simulink model "SPWH"  (R2022a)
settings: Solver=VariableStepAuto  StartTime=0.0  StopTime=84600  RelTol=1e-3
model workspace (MAT data in the model file):
  A = 10
  Eff = 0.8
  a = 5
  b = 5
undefined symbols (not defined in the file): B1, B49, csv, F1, F49, G1, G49, WeatherInput
libraries: slpidlib x2
settings Model: Creator=harry  LastModifiedBy=harry

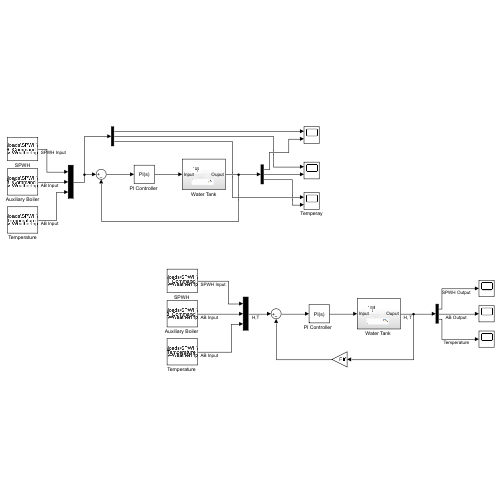
[thumbnail: Simulink's stored preview of the top-level diagram]
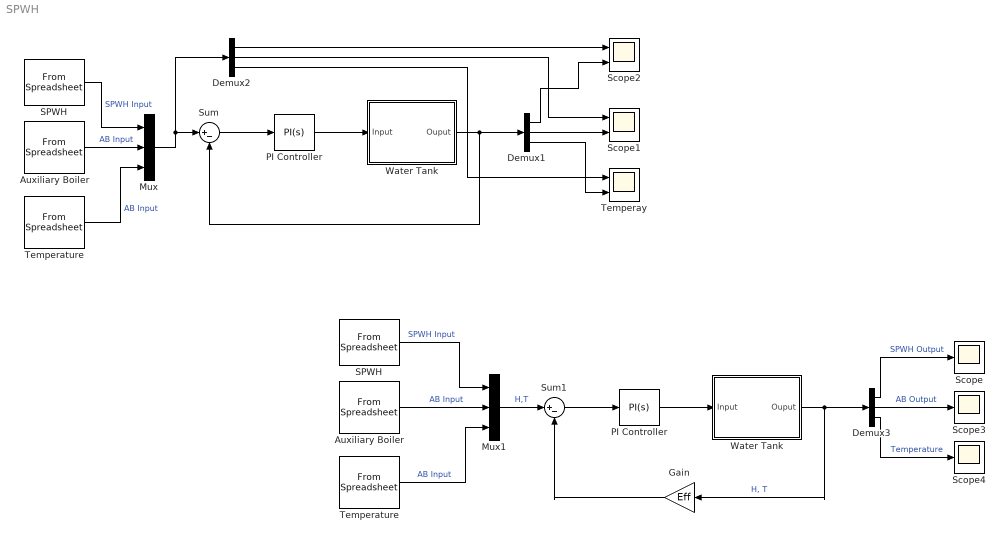
== system SPWH ==
  Auxiliary Boiler : FromSpreadsheet  FileName=C:\Users\harry\Downloads\SPWH\profiler-analyzer.xlsx  SheetName=csv-WeatherInput  Range=B1:B49,E1:E49
  "Auxiliary Boiler " : FromSpreadsheet  FileName=C:\Users\harry\Downloads\SPWH\profiler-analyzer.xlsx  SheetName=csv-WeatherInput  Range=B1:B49,E1:E49
  Demux1 : Demux  Outputs=3
  Demux2 : Demux  Outputs=3
  Demux3 : Demux  Outputs=3
  Gain : Gain  Gain=Eff
  Mux : Mux  Inputs=3
  Mux1 : Mux  Inputs=3
  "PI Controller " : slpidlib/PID Controller  Controller=PI  Form=Parallel  TimeDomain=Continuous-time  UseExternalTs=off  SampleTime=-1  IntegratorMethod=Forward Euler  FilterMethod=Forward Euler  ControllerParametersSource=internal  P=100  I=100  UseKiTs=off  D=0  N=100  UseFilter=on  TunerSelectOption=Transfer Function Based (PID Tuner App)  InitialConditionSource=internal  InitialConditionForIntegrator=0  InitialConditionForFilter=0  DifferentiatorICPrevScaledInput=0  ExternalReset=none  TrackingMode=off  Kt=1  LimitOutput=off  SatLimitsSource=internal  UpperSaturationLimit=inf  LowerSaturationLimit=-inf  LinearizeAsGain=on  AntiWindupMode=none  Kb=1  POutMin=[]  POutMax=[]  IOutMin=[]  IOutMax=[]  DOutMin=[]  DOutMax=[]  NOutMin=[]  NOutMax=[]  SumOutMin=[]  SumOutMax=[]  SaturationOutMin=[]  SaturationOutMax=[]  PParamMin=[]  PParamMax=[]  IParamMin=[]  IParamMax=[]  DParamMin=[]  DParamMax=[]  NParamMin=[]  NParamMax=[]  KbParamMin=[]  KbParamMax=[]  KtParamMin=[]  KtParamMax=[]  KbOutMin=[]  KbOutMax=[]  KtOutMin=[]  KtOutMax=[]  IntegratorOutMin=[]  IntegratorOutMax=[]  FilterOutMin=[]  FilterOutMax=[]  SumI1OutMin=[]  SumI1OutMax=[]  SumI2OutMin=[]  SumI2OutMax=[]  SumI3OutMin=[]  SumI3OutMax=[]  SumI4OutMin=[]  SumI4OutMax=[]  SumDOutMin=[]  SumDOutMax=[]  DifferentiatorOutMin=[]  DifferentiatorOutMax=[]  FilterDiffOutCoefMin=[]  FilterDiffOutCoefMax=[]  ReciprocalOutMin=[]  ReciprocalOutMax=[]  SumDenOutMin=[]  SumDenOutMax=[]  SumNumOutMin=[]  SumNumOutMax=[]  DivideOutMin=[]  DivideOutMax=[]  UdiffTsProdOutMin=[]  UdiffTsProdOutMax=[]  NTsProdOutMin=[]  NTsProdOutMax=[]  UintegralTsProdOutMin=[]  UintegralTsProdOutMax=[]  UngainTsProdOutMin=[]  UngainTsProdOutMax=[]  IntegratorContinuousStateAttributes=''  IntegratorStateMustResolveToSignalObject=off  IntegratorRTWStateStorageClass=Auto  FilterContinuousStateAttributes=''  FilterStateMustResolveToSignalObject=off  FilterRTWStateStorageClass=Auto  ParallelPVariant=InternalParameters  IdealPVariant=Disabled  IVariant=InternalParameters  DVariant=Disabled  IntegratorVariant=Continuous  SatVariant=Disabled  AWVariant=Passthrough  PCopyVariant=Disabled  TRVariant=Disabled  FdbkBlocksVariant=Forward  IdealPFdbkVariant=Disabled  SatFdbkVariant=Disabled  DerivativeFilterVariant=Disabled  NVariant=Disabled  NCopyVariant=Disabled_SignalSpec  FilterICVariant=Disabled  IntegratorICVariant=InternalICs  ExternalResetVariant=Disabled  TRSumVariant=Passthrough  SumFdbkVariant=Disabled  SumVariant=Sum_PI  TsampFilterVariant=InternalTs  TsampNgainVariant=Passthrough  TsampIntegralVariant=Passthrough  ExternalSaturationOutDataTypeStr=Inherit: Same as second input  aMode=0
  "PI Controller  " : slpidlib/PID Controller  Controller=PI  Form=Parallel  TimeDomain=Continuous-time  UseExternalTs=off  SampleTime=-1  IntegratorMethod=Forward Euler  FilterMethod=Forward Euler  ControllerParametersSource=internal  P=1  I=1  UseKiTs=off  D=0  N=100  UseFilter=on  TunerSelectOption=Transfer Function Based (PID Tuner App)  InitialConditionSource=internal  InitialConditionForIntegrator=0  InitialConditionForFilter=0  DifferentiatorICPrevScaledInput=0  ExternalReset=none  TrackingMode=off  Kt=1  LimitOutput=off  SatLimitsSource=internal  UpperSaturationLimit=inf  LowerSaturationLimit=-inf  LinearizeAsGain=on  AntiWindupMode=none  Kb=1  POutMin=[]  POutMax=[]  IOutMin=[]  IOutMax=[]  DOutMin=[]  DOutMax=[]  NOutMin=[]  NOutMax=[]  SumOutMin=[]  SumOutMax=[]  SaturationOutMin=[]  SaturationOutMax=[]  PParamMin=[]  PParamMax=[]  IParamMin=[]  IParamMax=[]  DParamMin=[]  DParamMax=[]  NParamMin=[]  NParamMax=[]  KbParamMin=[]  KbParamMax=[]  KtParamMin=[]  KtParamMax=[]  KbOutMin=[]  KbOutMax=[]  KtOutMin=[]  KtOutMax=[]  IntegratorOutMin=[]  IntegratorOutMax=[]  FilterOutMin=[]  FilterOutMax=[]  SumI1OutMin=[]  SumI1OutMax=[]  SumI2OutMin=[]  SumI2OutMax=[]  SumI3OutMin=[]  SumI3OutMax=[]  SumI4OutMin=[]  SumI4OutMax=[]  SumDOutMin=[]  SumDOutMax=[]  DifferentiatorOutMin=[]  DifferentiatorOutMax=[]  FilterDiffOutCoefMin=[]  FilterDiffOutCoefMax=[]  ReciprocalOutMin=[]  ReciprocalOutMax=[]  SumDenOutMin=[]  SumDenOutMax=[]  SumNumOutMin=[]  SumNumOutMax=[]  DivideOutMin=[]  DivideOutMax=[]  UdiffTsProdOutMin=[]  UdiffTsProdOutMax=[]  NTsProdOutMin=[]  NTsProdOutMax=[]  UintegralTsProdOutMin=[]  UintegralTsProdOutMax=[]  UngainTsProdOutMin=[]  UngainTsProdOutMax=[]  IntegratorContinuousStateAttributes=''  IntegratorStateMustResolveToSignalObject=off  IntegratorRTWStateStorageClass=Auto  FilterContinuousStateAttributes=''  FilterStateMustResolveToSignalObject=off  FilterRTWStateStorageClass=Auto  ParallelPVariant=InternalParameters  IdealPVariant=Disabled  IVariant=InternalParameters  DVariant=Disabled  IntegratorVariant=Continuous  SatVariant=Disabled  AWVariant=Passthrough  PCopyVariant=Disabled  TRVariant=Disabled  FdbkBlocksVariant=Forward  IdealPFdbkVariant=Disabled  SatFdbkVariant=Disabled  DerivativeFilterVariant=Disabled  NVariant=Disabled  NCopyVariant=Disabled_SignalSpec  FilterICVariant=Disabled  IntegratorICVariant=InternalICs  ExternalResetVariant=Disabled  TRSumVariant=Passthrough  SumFdbkVariant=Disabled  SumVariant=Sum_PI  TsampFilterVariant=InternalTs  TsampNgainVariant=Passthrough  TsampIntegralVariant=Passthrough  ExternalSaturationOutDataTypeStr=Inherit: Same as second input  aMode=0
  SPWH : FromSpreadsheet  FileName=C:\Users\harry\Downloads\SPWH\profiler-analyzer.xlsx  SheetName=csv-WeatherInput  Range=B1:B49,F1:F49
  "SPWH " : FromSpreadsheet  FileName=C:\Users\harry\Downloads\SPWH\profiler-analyzer.xlsx  SheetName=csv-WeatherInput  Range=B1:B49,F1:F49
  Scope : Scope
  Scope1 : Scope  NumInputPorts=2
  Scope2 : Scope  NumInputPorts=2
  Scope3 : Scope
  Scope4 : Scope
  Sum : Sum  Inputs=|+-
  Sum1 : Sum  Inputs=|+-
  Temperature : FromSpreadsheet  FileName=C:\Users\harry\Downloads\SPWH\profiler-analyzer.xlsx  SheetName=csv-WeatherInput  Range=B1:B49,G1:G49
  "Temperature " : FromSpreadsheet  FileName=C:\Users\harry\Downloads\SPWH\profiler-analyzer.xlsx  SheetName=csv-WeatherInput  Range=B1:B49,G1:G49
  Temperay : Scope  NumInputPorts=2
  Water Tank : Subsystem
  "Water Tank " : Subsystem
  wires:
  Water Tank/1(Ouput) -> Demux1/1, Sum/2
  Auxiliary Boiler/1 -> Mux/2  "AB Input"
  SPWH/1 -> Mux/1  "SPWH Input"
  Mux/1 -> Demux2/1, Sum/1
  Sum/1 -> "PI Controller "/1
  "PI Controller "/1 -> Water Tank/1("Input ")
  Demux1/1 -> Scope2/2
  Demux1/2 -> Scope1/2
  Demux2/1 -> Scope2/1
  Demux2/3 -> Temperay/1
  Temperature/1 -> Mux/3  "AB Input"
  Demux2/2 -> Scope1/1
  Demux1/3 -> Temperay/2
  Demux3/3 -> Scope4/1  "Temperature"
  Sum1/1 -> "PI Controller  "/1
  "Water Tank "/1(Ouput) -> Demux3/1, Gain/1  "H, T"
  "PI Controller  "/1 -> "Water Tank "/1("Input ")
  "Temperature "/1 -> Mux1/3  "AB Input"
  Demux3/2 -> Scope3/1  "AB Output"
  Demux3/1 -> Scope/1  "SPWH Output"
  "Auxiliary Boiler "/1 -> Mux1/2  "AB Input"
  "SPWH "/1 -> Mux1/1  "SPWH Input"
  Mux1/1 -> Sum1/1  "H,T"
  Gain/1 -> Sum1/2

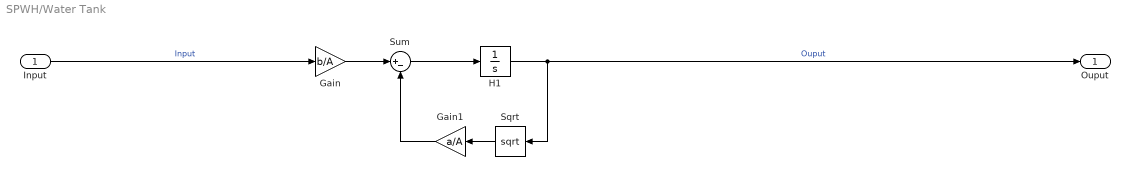
== system SPWH/Water Tank ==
  "Input " : Inport
  Gain : Gain  Gain=b/A
  Gain1 : Gain  Gain=a/A
  H1 : Integrator  InitialCondition=3  LimitOutput=on  LowerSaturationLimit=0
  Sqrt : Sqrt
  Sum : Sum  Inputs=|+-
  Ouput : Outport
  wires:
  Gain1/1 -> Sum/2
  "Input "/1 -> Gain/1  "Input"
  H1/1 -> Sqrt/1, Ouput/1  "Ouput"
  Gain/1 -> Sum/1
  Sum/1 -> H1/1
  Sqrt/1 -> Gain1/1

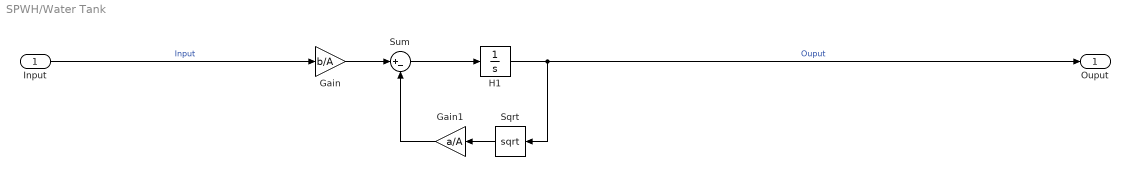
== system SPWH/Water Tank  ==
  "Input " : Inport
  Gain : Gain  Gain=b/A
  Gain1 : Gain  Gain=a/A
  H1 : Integrator  InitialCondition=3  LimitOutput=on  LowerSaturationLimit=0
  Sqrt : Sqrt
  Sum : Sum  Inputs=|+-
  Ouput : Outport
  wires:
  Gain1/1 -> Sum/2
  "Input "/1 -> Gain/1  "Input"
  H1/1 -> Sqrt/1, Ouput/1  "Ouput"
  Gain/1 -> Sum/1
  Sum/1 -> H1/1
  Sqrt/1 -> Gain1/1
